simulink model "SCARA_TS60"  (R2017a)
settings: Solver=FixedStepAuto  StartTime=0.0  StopTime=tmax  FixedStep=dt  RelTol=1e-1
values from neighbouring files (symbols this model uses):
  C1 = 0    [Initialisation_Interface_SCARA.m]    (also in SCARA_TS60_Interface.m = 1)
  C2 = 0    [Initialisation_Interface_SCARA.m]
  C3 = 0    [Initialisation_Interface_SCARA.m]    (also in SCARA_TS60_Interface.m = 1)
  C4 = 0    [Initialisation_Interface_SCARA.m]    (also in SCARA_TS60_Interface.m = 1)
libraries: fuzblock x3, roblocks1 x1
settings Model: Creator=El Rey  LastModifiedBy=El Rey

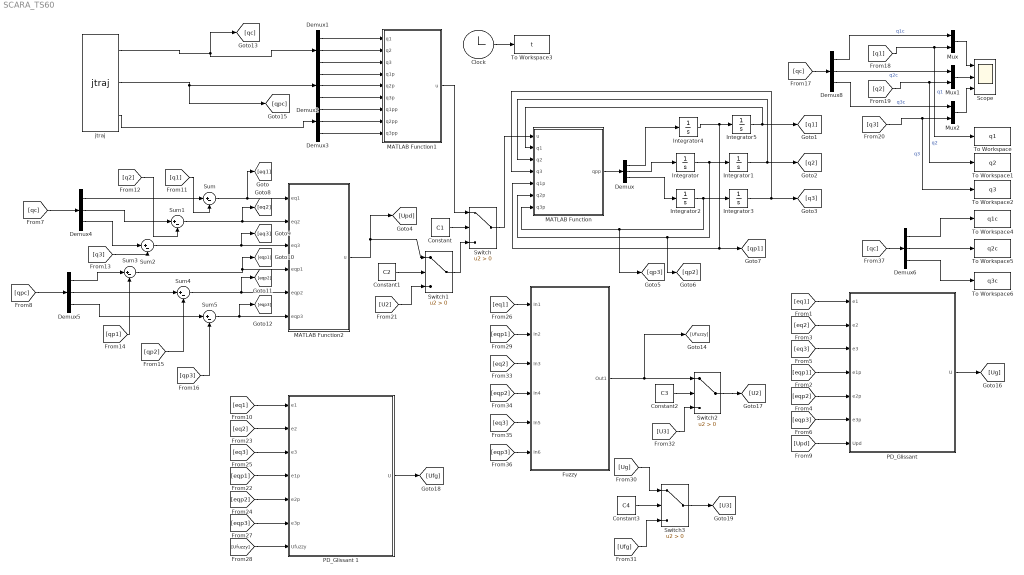
== system SCARA_TS60 ==
  Clock : Clock
  Constant : Constant  Value=C1
  Constant1 : Constant  Value=C2
  Constant2 : Constant  Value=C3
  Constant3 : Constant  Value=C4
  Demux{,1..6,8} (8 alike) : Demux  Outputs=3
  Fuzzy : Subsystem
  Integrator : Integrator  IgnoreLimit=on
  Integrator{1..3,5} (4 alike) : Integrator
  Integrator4 : Integrator  IgnoreLimit=on
  MATLAB Function : MATLAB Function  TreatAsAtomicUnit=on
  MATLAB Function1 : MATLAB Function  TreatAsAtomicUnit=on
  MATLAB Function2 : MATLAB Function  TreatAsAtomicUnit=on
  Mux : Mux  Inputs=2
  Mux1 : Mux  Inputs=2
  Mux2 : Mux  Inputs=2
  "PD_Glissant " : MATLAB Function  TreatAsAtomicUnit=on
  PD_Glissant 1 : MATLAB Function  TreatAsAtomicUnit=on
  Scope : Scope  NumInputPorts=3
  Sum{,1..5} (6 alike) : Sum  Inputs=|+-
  Switch{,1..3} (4 alike) : Switch  Criteria=u2 > Threshold
  To Workspace : ToWorkspace  VariableName=q1  SampleTime=-1
  To Workspace1 : ToWorkspace  VariableName=q2  SampleTime=-1
  To Workspace2 : ToWorkspace  VariableName=q3  SampleTime=-1
  To Workspace3 : ToWorkspace  VariableName=t  SampleTime=-1
  To Workspace4 : ToWorkspace  VariableName=q1c  SampleTime=-1
  To Workspace5 : ToWorkspace  VariableName=q2c  SampleTime=-1
  To Workspace6 : ToWorkspace  VariableName=q3c  SampleTime=-1
  jtraj : roblocks1/Toolbox/jtraj  q0=q0  qf=qf  tmax=tmax  ts=dt
  wires:
  Sum2/1 -> [eq3], MATLAB Function2/3(eq3)
  Sum5/1 -> [eqp3], MATLAB Function2/6(eqp3)
  Sum1/1 -> [eq2], MATLAB Function2/2(eq2)
  Sum4/1 -> [eqp2], MATLAB Function2/5(eqp2)
  Demux3/1 -> MATLAB Function1/7(q1pp)
  Sum3/1 -> [eqp1], MATLAB Function2/4(eqp1)
  Demux/1 -> Integrator4/1
  Switch/1 -> MATLAB Function/1(u)
  Demux/2 -> Integrator/1
  Demux1/3 -> MATLAB Function1/3(q3)
  Demux3/2 -> MATLAB Function1/8(q2pp)
  Mux2/1 -> Scope/3
  Demux2/2 -> MATLAB Function1/5(q2p)
  Integrator5/1 -> [q1], MATLAB Function/2(q1)
  Mux1/1 -> Scope/2
  Demux1/2 -> MATLAB Function1/2(q2)
  Demux2/1 -> MATLAB Function1/4(q1p)
  Integrator3/1 -> [q3], MATLAB Function/4(q3)
  Integrator1/1 -> [q2], MATLAB Function/3(q2)
  Sum/1 -> [eq1], MATLAB Function2/1(eq1)
  Demux1/1 -> MATLAB Function1/1(q1)
  Integrator/1 -> [qp2], MATLAB Function/6(q2p), Integrator1/1
  Demux/3 -> Integrator2/1
  Mux/1 -> Scope/1
  Demux2/3 -> MATLAB Function1/6(q3p)
  MATLAB Function/1(qpp) -> Demux/1
  Demux3/3 -> MATLAB Function1/9(q3pp)
  Integrator2/1 -> Integrator3/1, [qp3], MATLAB Function/7(q3p)
  [qc] -> Demux4/1
  Demux4/3 -> Sum2/1
  Demux4/2 -> Sum1/1
  Demux4/1 -> Sum/1
  [qpc] -> Demux5/1
  Demux5/1 -> Sum3/1
  Demux5/2 -> Sum4/1
  Demux5/3 -> Sum5/1
  [q1] -> Sum/2
  [q2] -> Sum1/2
  [q3] -> Sum2/2
  [qp3] -> Sum5/2
  [qp2] -> Sum4/2
  [qp1] -> Sum3/2
  [qc] -> Demux8/1
  Demux8/1 -> Mux/1  "q1c"
  Demux8/2 -> Mux1/1  "q2c"
  Demux8/3 -> Mux2/1  "q3c"
  [q1] -> To Workspace/1, Mux/2  "q1"
  [q2] -> To Workspace1/1, Mux1/2  "q2"
  [q3] -> To Workspace2/1, Mux2/2  "q3"
  "PD_Glissant "/1(U) -> [Ug]
  MATLAB Function2/1(u) -> Switch1/1, [Upd]
  [U2] -> Switch1/3
  Integrator4/1 -> MATLAB Function/5(q1p), [qp1], Integrator5/1
  [U3] -> Switch2/3
  Switch2/1 -> [U2]
  [eq1] -> Fuzzy/1(In1)
  [eqp1] -> Fuzzy/2(In2)
  [eq2] -> Fuzzy/3(In3)
  [eqp2] -> Fuzzy/4(In4)
  [eq3] -> Fuzzy/5(In5)
  [eqp3] -> Fuzzy/6(In6)
  Fuzzy/1(Out1) -> Switch2/1, [Ufuzzy]
  [eq1] -> "PD_Glissant "/1(e1)
  [eq2] -> "PD_Glissant "/2(e2)
  [eq3] -> "PD_Glissant "/3(e3)
  [eqp2] -> "PD_Glissant "/5(e2p)
  [eqp1] -> "PD_Glissant "/4(e1p)
  [eqp3] -> "PD_Glissant "/6(e3p)
  [Upd] -> "PD_Glissant "/7(Upd)
  [Ufuzzy] -> PD_Glissant 1/7(Ufuzzy)
  [eqp3] -> PD_Glissant 1/6(e3p)
  [eqp1] -> PD_Glissant 1/4(e1p)
  [eqp2] -> PD_Glissant 1/5(e2p)
  [eq3] -> PD_Glissant 1/3(e3)
  [eq2] -> PD_Glissant 1/2(e2)
  [eq1] -> PD_Glissant 1/1(e1)
  PD_Glissant 1/1(U) -> [Ufg]
  [Ug] -> Switch3/1
  [Ufg] -> Switch3/3
  Switch3/1 -> [U3]
  MATLAB Function1/1(u) -> Switch/1
  Switch1/1 -> Switch/3
  Constant/1 -> Switch/2
  Constant1/1 -> Switch1/2
  Constant2/1 -> Switch2/2
  Constant3/1 -> Switch3/2
  Clock/1 -> To Workspace3/1
  [qc] -> Demux6/1
  Demux6/2 -> To Workspace5/1
  Demux6/3 -> To Workspace6/1
  Demux6/1 -> To Workspace4/1
  jtraj/1 -> Demux1/1, [qc]
  jtraj/2 -> Demux2/1, [qpc]
  jtraj/3 -> Demux3/1

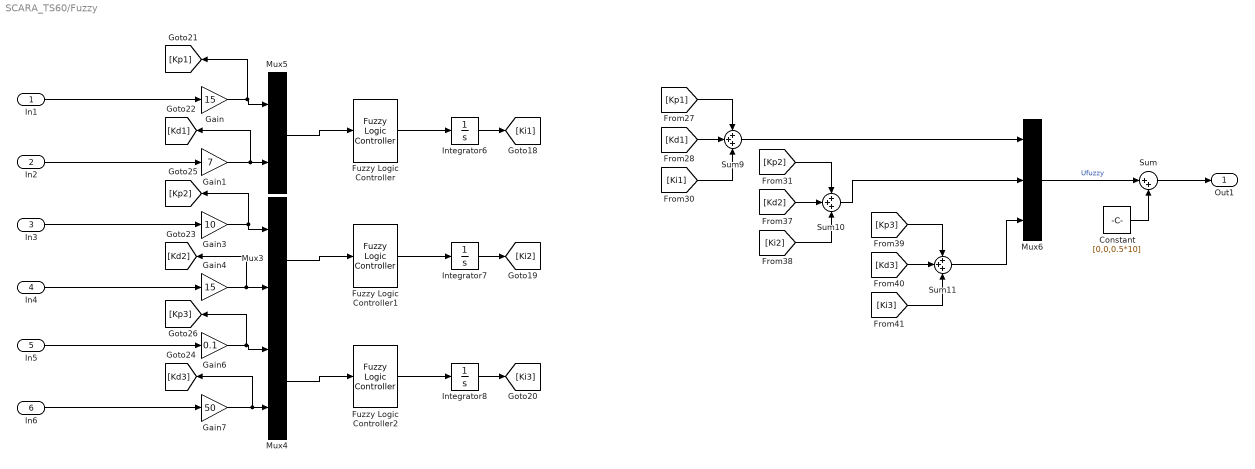
== system SCARA_TS60/Fuzzy ==
  In1 : Inport
  In2 : Inport  Port=2
  In3 : Inport  Port=3
  In4 : Inport  Port=4
  In5 : Inport  Port=5
  In6 : Inport  Port=6
  Constant : Constant  Value=[0,0,0.5*10]
  Fuzzy Logic Controller : fuzblock/Fuzzy Logic  Controller  fis='SCARA_FUZZY.fis'
  Fuzzy Logic Controller1 : fuzblock/Fuzzy Logic  Controller  fis='SCARA_FUZZY.fis'
  Fuzzy Logic Controller2 : fuzblock/Fuzzy Logic  Controller  fis='SCARA_FUZZY.fis'
  Gain : Gain  Gain=15
  Gain1 : Gain  Gain=7
  Gain3 : Gain  Gain=10
  Gain4 : Gain  Gain=15
  Gain6 : Gain  Gain=0.1
  Gain7 : Gain  Gain=50
  Integrator6 : Integrator
  Integrator7 : Integrator
  Integrator8 : Integrator
  Mux3 : Mux  Inputs=2
  Mux4 : Mux  Inputs=2
  Mux5 : Mux  Inputs=2
  Mux6 : Mux  Inputs=3
  Sum : Sum  Inputs=|++
  Sum10 : Sum  Inputs=+++
  Sum11 : Sum  Inputs=+++
  Sum9 : Sum  Inputs=+++
  Out1 : Outport
  wires:
  Mux5/1 -> Fuzzy Logic Controller/1
  In2/1 -> Gain1/1
  Fuzzy Logic Controller/1 -> Integrator6/1
  In1/1 -> Gain/1
  Gain4/1 -> [Kd2], Mux3/2
  Fuzzy Logic Controller1/1 -> Integrator7/1
  Mux3/1 -> Fuzzy Logic Controller1/1
  Mux4/1 -> Fuzzy Logic Controller2/1
  In4/1 -> Gain4/1
  Gain3/1 -> [Kp2], Mux3/1
  Gain7/1 -> [Kd3], Mux4/2
  Gain6/1 -> [Kp3], Mux4/1
  Fuzzy Logic Controller2/1 -> Integrator8/1
  In5/1 -> Gain6/1
  In6/1 -> Gain7/1
  Gain/1 -> [Kp1], Mux5/1
  In3/1 -> Gain3/1
  Gain1/1 -> [Kd1], Mux5/2
  Integrator7/1 -> [Ki2]
  [Ki3] -> Sum11/3
  [Ki1] -> Sum9/3
  [Ki2] -> Sum10/3
  Sum10/1 -> Mux6/2
  [Kp3] -> Sum11/1
  [Kd3] -> Sum11/2
  Integrator8/1 -> [Ki3]
  [Kd2] -> Sum10/2
  [Kp1] -> Sum9/1
  [Kp2] -> Sum10/1
  [Kd1] -> Sum9/2
  Sum9/1 -> Mux6/1
  Sum11/1 -> Mux6/3
  Integrator6/1 -> [Ki1]
  Sum/1 -> Out1/1
  Mux6/1 -> Sum/1  "Ufuzzy"
  Constant/1 -> Sum/2

== matlab function SCARA_TS60/MATLAB Function1 ==
  data: q1 input; u output; q2 input; q3 input; q1p input; q2p input; q3p input; q1pp input; q2pp input; q3pp input
function u = SCARA_MDD(q1,q2,q3,q1p,q2p,q3p,q1pp,q2pp,q3pp)
%---definition des constantes---%

qpp=zeros(3,1);qp=zeros(3,1);q=zeros(3,1);
q(1,1)=q1;q(2,1)=q2;q(3,1)=q3;
qp(1,1)=q1p;qp(2,1)=q2p;qp(3,1)=q3p;
qpp(1,1)=q1pp;qpp(2,1)=q2pp;qpp(3,1)=q3pp;
m0=19.5;m1=8;m2=6;m3=0.5;
d0=0.65;d1=0.4;d2=0.3;d3=0.3;
I0=1.0298;I1=0.16;I2=0.0675;I3=0.0056;
g=10;
%--------------------------------%
M=zeros(3);
M(1,1)=I1+I2+I3+(m3+0.25*m1+m2)*d1^2+(0.25*m2+m3)*d2^2+(2*m3+m2)*d1*d2*cos(q2);
M(1,2)=I2+I3+(0.25*m2+m3)*d2^2+(0.5*m2+m3)*d1*d2*cos(q2); %
M(1,3)=0; %
M(2,1)=M(1,2); %
M(2,2)=I2+I3+(0.25*m2+m3)*d2^2; %
M(2,3)=0; %
M(3,1)=M(1,3); %
M(3,2)=M(2,3); %
M(3,3)=m3;
N=zeros(3); %
N(1,1)=-0.5*d1*d2*sin(q2)*(2*m3+m2)*q2p; %
N(1,2)=-0.5*d1*d2*sin(q2)*(2*m3+m2)*(q1p+q2p); %
N(1,3)=0; %
N(2,1)=-0.5*d1*d2*sin(q2)*(2*m3+m2)*(q1p+q2p); %
N(2,2)=-0.5*d1*d2*sin(q2)*(2*m3+m2)*q1p; %
N(2,3)=0; %
N(3,1)=0; %
N(3,2)=0; %
N(3,3)=0;
%------ Vecteur de gravité ----------------------%
G=zeros(3,1); %
G(1)=0; %
G(2)=0; %
G(3)=m3*g;
%--reponse de la forme qpp = (1/M)*(u-N*qp-G)-----%
u = M*qpp+N*qp+G;

== matlab function SCARA_TS60/MATLAB Function ==
  data: u input; qpp output; q1 input; q2 input; q3 input; q1p input; q2p input; q3p input
function qpp = SCARA_MDI(u,q1,q2,q3,q1p,q2p,q3p)
%---definition des constantes---%
qp=zeros(3,1);q=zeros(3,1);
qp(1,1)=q1p;qp(2,1)=q2p;qp(3,1)=q3p;
m0=19.5;
m1=8;
m2=6; 
m3=0.5;
d0=0.65;
d1=0.4;
d2=0.3;
d3=0.3;%%0.3
I0=1.0298;
I1=0.16;
I2=0.0675;
I3=0.0056;
g=10;
%--------------------------------%
M=zeros(3);
M(1,1)=I1+I2+I3+(m3+0.25*m1+m2)*d1^2+(0.25*m2+m3)*d2^2+(2*m3+m2)*d1*d2*cos(q2);
M(1,2)=I2+I3+(0.25*m2+m3)*d2^2+(0.5*m2+m3)*d1*d2*cos(q2); %
M(1,3)=0; %
M(2,1)=M(1,2); %
M(2,2)=I2+I3+(0.25*m2+m3)*d2^2; %
M(2,3)=0; %
M(3,1)=M(1,3); %
M(3,2)=M(2,3); %
M(3,3)=m3;
N=zeros(3); %
N(1,1)=-0.5*d1*d2*sin(q2)*(2*m3+m2)*q2p; %
N(1,2)=-0.5*d1*d2*sin(q2)*(2*m3+m2)*(q1p+q2p); %
N(1,3)=0; %
N(2,1)=-0.5*d1*d2*sin(q2)*(2*m3+m2)*(q1p+q2p); %
N(2,2)=-0.5*d1*d2*sin(q2)*(2*m3+m2)*q1p; %
N(2,3)=0; %
N(3,1)=0; %
N(3,2)=0; %
N(3,3)=0;
%------ Vecteur de gravité ----------------------%
G=zeros(3,1); %
G(1)=0; %
G(2)=0; %
G(3)=m3*g;
%--reponse de la forme qpp = (1/M)*(u-N*qp-G)-----%
qpp = pinv(M)*(u-N*qp-G);

== matlab function SCARA_TS60/MATLAB Function2 ==
  data: eq1 input; u output; eq2 input; eq3 input; eqp1 input; eqp2 input; eqp3 input
function u = com_PD(eq1,eq2,eq3,eqp1,eqp2,eqp3)
eq=zeros(3,1);eqp=zeros(3,1);
eq(1,1)=eq1;eq(2,1)=eq2;eq(3,1)=eq3;
eqp(1,1)=eqp1;eqp(2,1)=eqp2;eqp(3,1)=eqp3;
m0=19.5;m1=8;m2=6;m3=0.5;
g=10;
%------ Vecteur de gravité ----------------------%
G=zeros(3,1); %
G(1)=0; %
G(2)=0; %
G(3)=m3*g;
Kp = diag([15,15,0.10]);
Kd=diag([7,10,50]);
u = Kp*eq+Kd*eqp+G;

== matlab function SCARA_TS60/PD_Glissant  ==
  data: e1 input; U output; e2 input; e3 input; e1p input; e2p input; e3p input; Upd input
function U = Mode_Glissant(e1,e2,e3,e1p,e2p,e3p,Upd)
%--reponse de la forme U = Ueq + dU -----%
K=0.15;L=1;% K=0.00001;L=1; avec Ueq=U
ep=zeros(3,1);
ep(1,1)=e1p;
ep(2,1)=e2p;
ep(3,1)=e3p;
e=zeros(3,1);
e(1,1)=e1;
e(2,1)=e2;
e(3,1)=e3;
s=ep+L*e;

dU = -K*sign(s);
U = Upd + dU;

== matlab function SCARA_TS60/PD_Glissant 1 ==
  data: e1 input; U output; e2 input; e3 input; e1p input; e2p input; e3p input; Ufuzzy input
function U = Mode_Glissant_Floue(e1,e2,e3,e1p,e2p,e3p,Ufuzzy)
%--reponse de la forme U = Ueq + dU -----%
K=0.15;L=1;% K=0.00001;L=1; avec Ueq=U
ep=zeros(3,1);
ep(1,1)=e1p;
ep(2,1)=e2p;
ep(3,1)=e3p;
e=zeros(3,1);
e(1,1)=e1;
e(2,1)=e2;
e(3,1)=e3;
s=ep+L*e;

dU = -K*sign(s);
U = Ufuzzy + dU;
